simulink model "Malha_fechada_2016"  (R2022b)
settings: Solver=FixedStepAuto  StartTime=0.0  StopTime=250.0  RelTol=1e-3
values from neighbouring files (symbols this model uses):
  den = [6000 1100 60 1]    [Analisa_malha_aberta.m]    (also in Analisa_malha_fechada.m)
  num = 15    [Analisa_malha_aberta.m]    (also in Analisa_malha_fechada.m)
settings Model: Creator=mluser  LastModifiedBy=mluser
settings SolverCC: AlgebraicLoopSolver=TrustRegion
settings DebuggingCC: ArithmeticOperatorsInVariantConditions=warning
settings SFSimCC: CustomCodeUndefinedFunction=UseInterfaceOnly
settings CodeAppCC: StateflowObjectComments=on

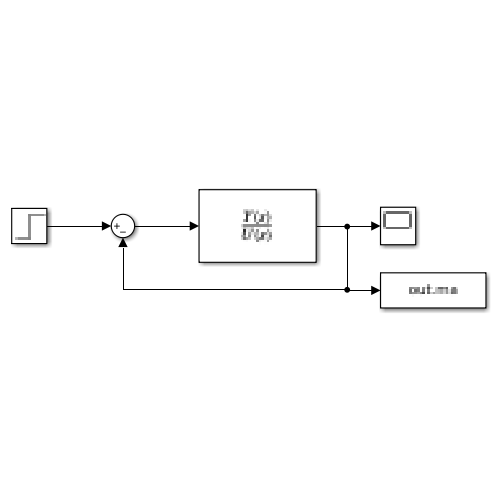
[thumbnail: Simulink's stored preview of the top-level diagram]
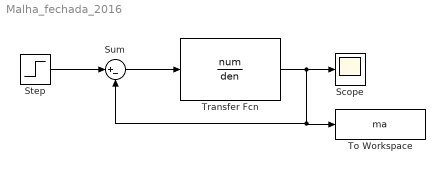
== system Malha_fechada_2016 ==
  Scope : Scope
  Step : Step  SampleTime=0
  Sum : Sum  Inputs=|+-
  To Workspace : ToWorkspace  VariableName=ma  SampleTime=-1
  Transfer Fcn : TransferFcn  Numerator=num  Denominator=den
  wires:
  Transfer Fcn/1 -> Sum/2, To Workspace/1, Scope/1
  Sum/1 -> Transfer Fcn/1
  Step/1 -> Sum/1
